simulink model "newfinal"  (R2022a)
settings: Solver=VariableStepAuto  StartTime=0.0  StopTime=time_to_simulate  RelTol=1e-3
model workspace (MAT data in the model file):
  Lm = 0.126
  Rm = 146.7889
  windingl = [0.3203609 0.3203609 0.3203609 0.000464923 0.000464923 0.000464923]
  windingr = [0.046115 0.046115 0.046115 6.692455e-05 6.692455e-05 6.692455e-05]
undefined symbols (not defined in the file): f, L1Aa, L1Ab, L1Ac, L1Ba, L1Bb, L1Bc, L1Ca, L1Cb, L1Cc, L2Aa, L2Ab, L2Ac, L2Ba, L2Bb, L2Bc, L2Ca, L2Cb, L2Cc, R1Aa, R1Ab, R1Ac, R1Ba, R1Bb, R1Bc, R1Ca, R1Cb, R1Cc, R2Aa, R2Ab, R2Ac, R2Ba, R2Bb, R2Bc, R2Ca, R2Cb, R2Cc, Sph, Ts, U1Aa, U1Ab, U1Ac, U1Ba, U1Bb, U1Bc, U1Ca, U1Cb, U1Cc, U2Aa, U2Ab, U2Ac, U2Ba, U2Bb, U2Bc, U2Ca, U2Cb, U2Cc, V1
libraries: spsBreakerLib x18, spsCurrentMeasurementLib x12, spsVoltageMeasurementLib x6, spsMultiWindingTransformerLib x3, spsGroundLib x2, spsThreePhaseParallelRLCLoadLib x1, spsThreePhaseSourceLib x1, spspowerguiLib x1
settings Model: Creator=Edwin  LastModifiedBy=Edwin
settings DebuggingCC: UnconnectedInputMsg=warning  UnconnectedOutputMsg=warning  UnconnectedLineMsg=warning
settings RTWCC: DLArmComputeVersion=19.05

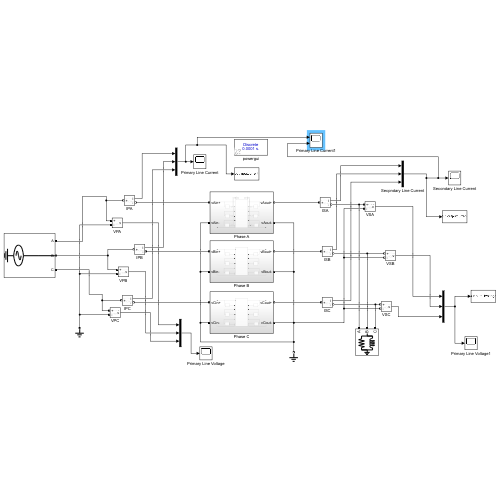
[thumbnail: Simulink's stored preview of the top-level diagram]
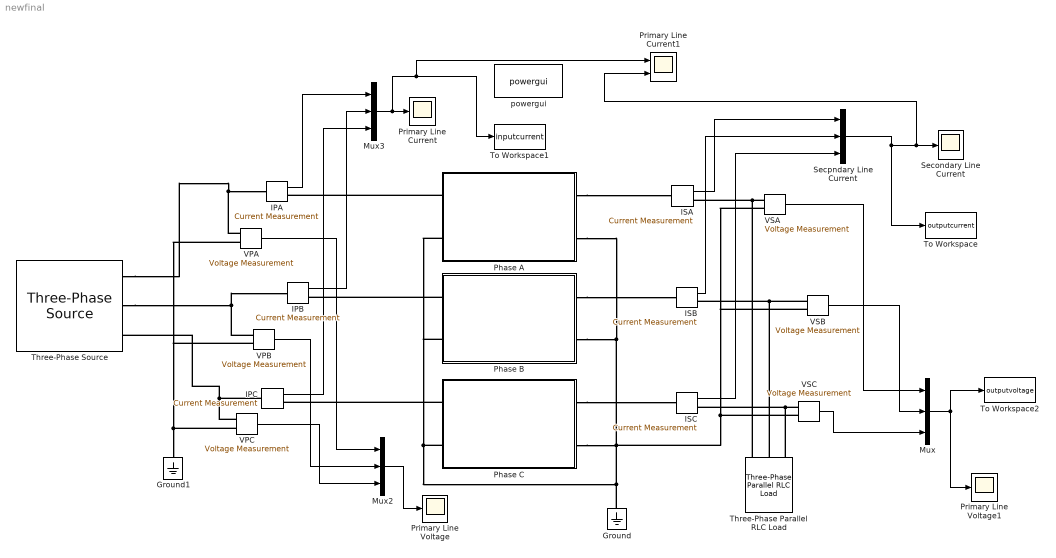
== system newfinal ==
  Ground : spsGroundLib/Ground  LConnTagsString=a
  Ground1 : spsGroundLib/Ground  LConnTagsString=a
  IPA : spsCurrentMeasurementLib/Current Measurement  PhasorSimulation=off  OutputType=Complex  PSBequivalent=0
  IPB : spsCurrentMeasurementLib/Current Measurement  PhasorSimulation=off  OutputType=Complex  PSBequivalent=0
  IPC : spsCurrentMeasurementLib/Current Measurement  PhasorSimulation=off  OutputType=Complex  PSBequivalent=0
  ISA : spsCurrentMeasurementLib/Current Measurement  PhasorSimulation=off  OutputType=Complex  PSBequivalent=0
  ISB : spsCurrentMeasurementLib/Current Measurement  PhasorSimulation=off  OutputType=Complex  PSBequivalent=0
  ISC : spsCurrentMeasurementLib/Current Measurement  PhasorSimulation=off  OutputType=Complex  PSBequivalent=0
  Mux : Mux  Inputs=3
  Mux2 : Mux  Inputs=3
  Mux3 : Mux  Inputs=3
  Phase A : Subsystem
  Phase B : Subsystem
  Phase C : Subsystem
  Primary Line Current : Scope
  Primary Line Current1 : Scope  NumInputPorts=2
  Primary Line Voltage : Scope
  Primary Line Voltage1 : Scope
  Secondary Line Current : Scope
  Secpndary Line Current : Mux  Inputs=3
  Three-Phase Parallel RLC Load : spsThreePhaseParallelRLCLoadLib/Three-Phase Parallel RLC Load  LConnTagsString=A|B|C  Configuration=Y (grounded)  NominalVoltage=V2ph  Vabc=[1e3 1e3 1e3]  Vabcp=[1e3 1e3 1e3]  NominalFrequency=f  UnbalancedPower=off  ActivePower=Pload  InductivePower=Qload  CapacitivePower=0  Pabc=[10e3 9e3 11e3]  QLabc=[100 90 110]  QCabc=[100 90 110]  Pabcp=[10e3 9e3 11e3]  QLabcp=[100 90 110]  QCabcp=[100 90 110]  Measurements=None  LoadType=constant Z
  Three-Phase Source : spsThreePhaseSourceLib/Three-Phase Source  InternalConnection=Yg  VoltagePhases=off  Voltage=V1  PhaseAngle=0  Voltage_phases=[10.5e3 10.5e3 10.5e3]/sqrt(3)  PhaseAngles_phases=[0 -120 +120]  Frequency=f  NonIdealSource=off  SpecifyImpedance=off  Resistance=0.8929  Inductance=16.58e-3  ShortCircuitLevel=100e6  BaseVoltage=25e3  XRratio=7  BusType=swing  Pref=10e3  Qref=0  Prefabc=[10e3, 10e3, 10e3]  Qrefabc=[0, 0, 0]  Qmin=-inf  Qmax=inf
  To Workspace : ToWorkspace  VariableName=outputcurrent  SampleTime=-1
  To Workspace1 : ToWorkspace  VariableName=inputcurrent  SampleTime=-1
  To Workspace2 : ToWorkspace  VariableName=outputvoltage  SampleTime=-1
  VPA : spsVoltageMeasurementLib/Voltage Measurement  PhasorSimulation=off  OutputType=Complex  PSBequivalent=0
  VPB : spsVoltageMeasurementLib/Voltage Measurement  PhasorSimulation=off  OutputType=Complex  PSBequivalent=0
  VPC : spsVoltageMeasurementLib/Voltage Measurement  PhasorSimulation=off  OutputType=Complex  PSBequivalent=0
  VSA : spsVoltageMeasurementLib/Voltage Measurement  PhasorSimulation=off  OutputType=Complex  PSBequivalent=0
  VSB : spsVoltageMeasurementLib/Voltage Measurement  PhasorSimulation=off  OutputType=Complex  PSBequivalent=0
  VSC : spsVoltageMeasurementLib/Voltage Measurement  PhasorSimulation=off  OutputType=Complex  PSBequivalent=0
  powergui : spspowerguiLib/powergui  Priority=1  SimulationMode=Discrete  SampleTime=Ts  frequency=60  Iterations=50  frequencyindice=50  Pbase=100e6  ErrMax=1e-4  UnitsV=kV  UnitsW=MW  buscounter=0  FunctionMessages=off  echomessages=off  EnableUseOfTLC=off  CurrentSourceSwitches=off  DisableSnubberDevices=off  DisableRonSwitches=off  DisableVfSwitches=off  DisplayEquations=off  AutomaticDiscreteSolvers=off  SolverType=Tustin/Backward Euler (TBE)  Interpol=off  ExternalGateDelay=off  methode=off  Ts=100  x0status=blocks  SPID=on  SwTol=0  HookPort=off  NonlinearTolerance=1e-4  nMaxIteration=100  ContinueOnMaxIteration=off  RestoreLinks=warning  ResistiveCurrentMeasurement=off  Frange=[0:2:500]  Ylog=off  Xlog=on  ShowGrid=off  save=off  variable=ZData  structure=0  ZoomFFT=off  StartTime=0.0  cycles=1  DisplayStyle=1  fundamental=60  FreqAxis=off  MaxFrequency=1000  frequencyindicesteady=1  RmsSteady=1  display=off
  wires:
  IPC/1 -> Mux3/3
  IPB/1 -> Mux3/2
  IPA/1 -> Mux3/1
  VPA/1 -> Mux2/1
  VPB/1 -> Mux2/2
  VPC/1 -> Mux2/3
  Mux3/1 -> Primary Line Current1/1, To Workspace1/1, Primary Line Current/1
  Mux2/1 -> Primary Line Voltage/1
  ISC/1 -> Secpndary Line Current/3
  ISB/1 -> Secpndary Line Current/2
  ISA/1 -> Secpndary Line Current/1
  VSA/1 -> Mux/1
  VSB/1 -> Mux/2
  VSC/1 -> Mux/3
  Secpndary Line Current/1 -> To Workspace/1, Primary Line Current1/2, Secondary Line Current/1
  Mux/1 -> To Workspace2/1, Primary Line Voltage1/1
  connections:
  Three-Phase Source/RConn1 -- VPA/LConn1 -- IPA/LConn1
  Three-Phase Source/RConn2 -- VPB/LConn1 -- IPB/LConn1
  IPC/LConn1 -- Three-Phase Source/RConn3 -- VPC/LConn1
  VPC/LConn2 -- VPA/LConn2 -- VPB/LConn2 -- Ground1/LConn1
  Phase A/LConn1 -- IPA/RConn1
  Phase B/LConn1 -- IPB/RConn1
  Phase C/LConn1 -- IPC/RConn1
  Phase A/RConn1 -- ISA/LConn1
  Phase B/RConn1 -- ISB/LConn1
  Phase C/RConn1 -- ISC/LConn1
  Ground/LConn1 -- Phase A/LConn2 -- Phase B/LConn2 -- Phase C/LConn2 -- Phase C/RConn2 -- VSC/LConn2 -- VSB/LConn2 -- VSA/LConn2 -- Phase B/RConn2 -- Phase A/RConn2
  VSC/LConn1 -- Three-Phase Parallel RLC Load/LConn3 -- ISC/RConn1
  VSB/LConn1 -- Three-Phase Parallel RLC Load/LConn2 -- ISB/RConn1
  VSA/LConn1 -- ISA/RConn1 -- Three-Phase Parallel RLC Load/LConn1

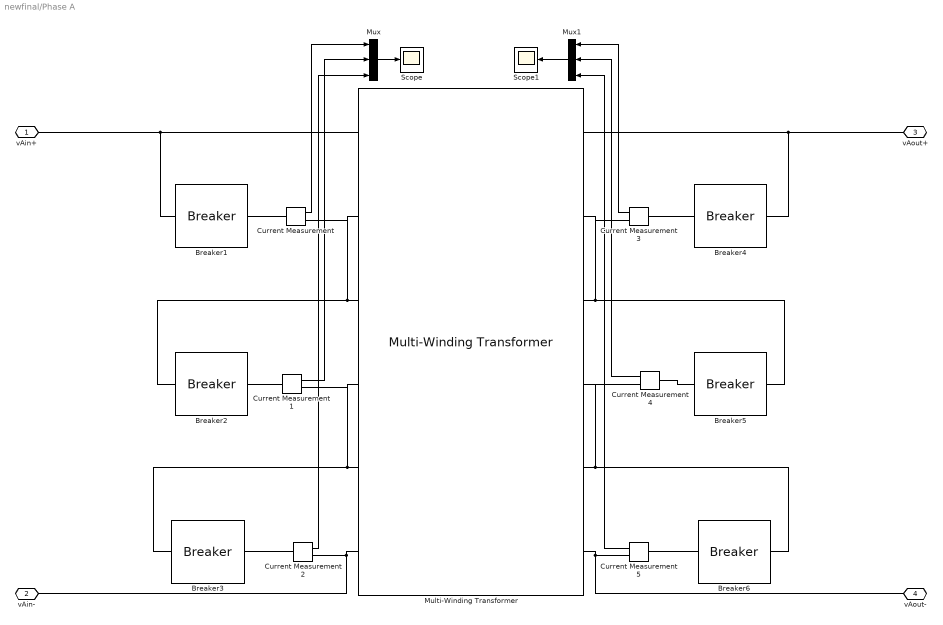
== system newfinal/Phase A ==
  Breaker1 : spsBreakerLib/Breaker  InitialState=0  SwitchingTimes=BreakerA1  External=off  BreakerResistance=0.01  SnubberResistance=1e6  SnubberCapacitance=inf  Measurements=Branch voltage and current  MoreParameters=on  NoBreakLoop=off
      settings: SourceProductBaseCode=PS
  Breaker2 : spsBreakerLib/Breaker  InitialState=0  SwitchingTimes=BreakerA2  External=off  BreakerResistance=0.01  SnubberResistance=1e6  SnubberCapacitance=inf  Measurements=Branch voltage and current  MoreParameters=on  NoBreakLoop=off
      settings: SourceProductBaseCode=PS
  Breaker3 : spsBreakerLib/Breaker  InitialState=0  SwitchingTimes=BreakerA3  External=off  BreakerResistance=0.01  SnubberResistance=1e6  SnubberCapacitance=inf  Measurements=Branch voltage and current  MoreParameters=on  NoBreakLoop=off
      settings: SourceProductBaseCode=PS
  Breaker4 : spsBreakerLib/Breaker  InitialState=0  SwitchingTimes=BreakerA4  External=off  BreakerResistance=0.01  SnubberResistance=1e6  SnubberCapacitance=inf  Measurements=Branch voltage and current  MoreParameters=on  NoBreakLoop=off
      settings: SourceProductBaseCode=PS
  Breaker5 : spsBreakerLib/Breaker  InitialState=0  SwitchingTimes=BreakerA5  External=off  BreakerResistance=0.01  SnubberResistance=1e6  SnubberCapacitance=inf  Measurements=Branch voltage and current  MoreParameters=on  NoBreakLoop=off
      settings: SourceProductBaseCode=PS
  Breaker6 : spsBreakerLib/Breaker  InitialState=0  SwitchingTimes=BreakerA6  External=off  BreakerResistance=0.01  SnubberResistance=1e6  SnubberCapacitance=inf  Measurements=Branch voltage and current  MoreParameters=on  NoBreakLoop=off
      settings: SourceProductBaseCode=PS
  Current Measurement{,1..5} (6 alike) : spsCurrentMeasurementLib/Current Measurement  PhasorSimulation=off  OutputType=Complex  PSBequivalent=0
  Multi-Winding Transformer : spsMultiWindingTransformerLib/Multi-Winding Transformer  LeftWindings=3  RightWindings=3  TappedWindings=no taps  NumberOfTaps=2  SetSaturation=off  Hysteresis=off  DataFile='hysteresis.mat'  Measurements=All measurements (V I Flux)  UNITS=SI  NominalPower=[Sph f]  NominalVoltages="[ U1Aa  U1Ab  U1Ac  U2Aa  U2Ab  U2Ac ]"  WindingResistances="[ R1Aa  R1Ab  R1Ac  R2Aa  R2Ab  R2Ac ]"  WindingInductances="[ L1Aa  L1Ab  L1Ac  L2Aa  L2Ab  L2Ac ]"  Rm=Rm  Lm=Lm  Saturation=[0 0;0.011719 56026;4.8828 70968]  SpecifyInitialFlux=off  InitialFlux=0  BreakLoop=off  DiscreteSolver=Trapezoidal iterative  DataType=on  TransfoNumber=1
      settings: SourceProductBaseCode=PS
  Mux : Mux  Inputs=3
  Mux1 : Mux  Inputs=3
  Scope : Scope
  Scope1 : Scope
  vAin+ : PMIOPort  Side=Left
  vAin- : PMIOPort  Port=2  Side=Left
  vAout+ : PMIOPort  Port=3  Side=Right
  vAout- : PMIOPort  Port=4  Side=Right
  wires:
  Current Measurement3/1 -> Mux1/1
  Current Measurement/1 -> Mux/1
  Current Measurement4/1 -> Mux1/2
  Current Measurement5/1 -> Mux1/3
  Current Measurement1/1 -> Mux/2
  Mux/1 -> Scope/1
  Current Measurement2/1 -> Mux/3
  Mux1/1 -> Scope1/1
  connections:
  Multi-Winding Transformer/LConn3 -- Breaker2/RConn1 -- Multi-Winding Transformer/LConn2 -- Current Measurement/RConn1
  Multi-Winding Transformer/RConn3 -- Multi-Winding Transformer/RConn2 -- Current Measurement3/RConn1 -- Breaker5/RConn1
  Multi-Winding Transformer/LConn5 -- Breaker3/RConn1 -- Multi-Winding Transformer/LConn4 -- Current Measurement1/RConn1
  Breaker4/RConn1 -- Multi-Winding Transformer/RConn1 -- vAout+/RConn1
  Current Measurement2/RConn1 -- vAin-/RConn1 -- Multi-Winding Transformer/LConn6
  Current Measurement5/RConn1 -- vAout-/RConn1 -- Multi-Winding Transformer/RConn6
  Multi-Winding Transformer/RConn5 -- Multi-Winding Transformer/RConn4 -- Current Measurement4/RConn1 -- Breaker6/RConn1
  Breaker1/RConn1 -- Multi-Winding Transformer/LConn1 -- vAin+/RConn1
  Current Measurement5/LConn1 -- Breaker6/LConn1
  Current Measurement2/LConn1 -- Breaker3/LConn1
  Current Measurement3/LConn1 -- Breaker4/LConn1
  Current Measurement/LConn1 -- Breaker1/LConn1
  Current Measurement4/LConn1 -- Breaker5/LConn1
  Current Measurement1/LConn1 -- Breaker2/LConn1

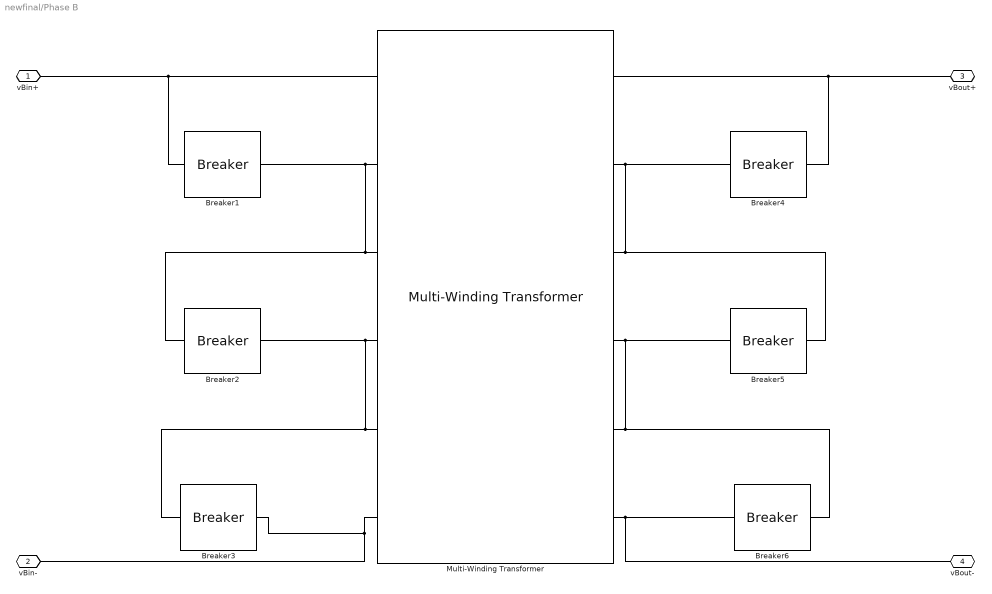
== system newfinal/Phase B ==
  Breaker1 : spsBreakerLib/Breaker  InitialState=0  SwitchingTimes=BreakerB1  External=off  BreakerResistance=0.01  SnubberResistance=1e6  SnubberCapacitance=inf  Measurements=Branch voltage and current  MoreParameters=on  NoBreakLoop=off
      settings: SourceProductBaseCode=PS
  Breaker2 : spsBreakerLib/Breaker  InitialState=0  SwitchingTimes=BreakerB2  External=off  BreakerResistance=0.01  SnubberResistance=1e6  SnubberCapacitance=inf  Measurements=Branch voltage and current  MoreParameters=on  NoBreakLoop=off
      settings: SourceProductBaseCode=PS
  Breaker3 : spsBreakerLib/Breaker  InitialState=0  SwitchingTimes=BreakerB3  External=off  BreakerResistance=0.01  SnubberResistance=1e6  SnubberCapacitance=inf  Measurements=Branch voltage and current  MoreParameters=on  NoBreakLoop=off
      settings: SourceProductBaseCode=PS
  Breaker4 : spsBreakerLib/Breaker  InitialState=0  SwitchingTimes=BreakerB4  External=off  BreakerResistance=0.01  SnubberResistance=1e6  SnubberCapacitance=inf  Measurements=Branch voltage and current  MoreParameters=on  NoBreakLoop=off
      settings: SourceProductBaseCode=PS
  Breaker5 : spsBreakerLib/Breaker  InitialState=0  SwitchingTimes=BreakerB5  External=off  BreakerResistance=0.01  SnubberResistance=1e6  SnubberCapacitance=inf  Measurements=Branch voltage and current  MoreParameters=on  NoBreakLoop=off
      settings: SourceProductBaseCode=PS
  Breaker6 : spsBreakerLib/Breaker  InitialState=0  SwitchingTimes=BreakerB6  External=off  BreakerResistance=0.01  SnubberResistance=1e6  SnubberCapacitance=inf  Measurements=Branch voltage and current  MoreParameters=on  NoBreakLoop=off
      settings: SourceProductBaseCode=PS
  Multi-Winding Transformer : spsMultiWindingTransformerLib/Multi-Winding Transformer  LeftWindings=3  RightWindings=3  TappedWindings=no taps  NumberOfTaps=2  SetSaturation=off  Hysteresis=off  DataFile='hysteresis.mat'  Measurements=All measurements (V I Flux)  UNITS=SI  NominalPower=[Sph f]  NominalVoltages="[ U1Ba  U1Bb  U1Bc  U2Ba  U2Bb  U2Bc ]"  WindingResistances="[ R1Ba  R1Bb  R1Bc  R2Ba  R2Bb  R2Bc ]"  WindingInductances="[ L1Ba  L1Bb  L1Bc  L2Ba  L2Bb  L2Bc ]"  Rm=Rm  Lm=Lm  Saturation=[0 0;0.011719 56026;4.8828 70968]  SpecifyInitialFlux=off  InitialFlux=0  BreakLoop=off  DiscreteSolver=Trapezoidal iterative  DataType=on  TransfoNumber=1
      settings: SourceProductBaseCode=PS
  vBin+ : PMIOPort  Side=Left
  vBin- : PMIOPort  Port=2  Side=Left
  vBout+ : PMIOPort  Port=3  Side=Right
  vBout- : PMIOPort  Port=4  Side=Right
  connections:
  Breaker1/LConn1 -- Multi-Winding Transformer/LConn2 -- Breaker2/RConn1 -- Multi-Winding Transformer/LConn3
  Breaker6/LConn1 -- Multi-Winding Transformer/RConn6 -- vBout-/RConn1
  Breaker4/RConn1 -- Multi-Winding Transformer/RConn1 -- vBout+/RConn1
  Multi-Winding Transformer/LConn5 -- Multi-Winding Transformer/LConn4 -- Breaker2/LConn1 -- Breaker3/RConn1
  Breaker4/LConn1 -- Multi-Winding Transformer/RConn2 -- Breaker5/RConn1 -- Multi-Winding Transformer/RConn3
  vBin-/RConn1 -- Breaker3/LConn1 -- Multi-Winding Transformer/LConn6
  Breaker5/LConn1 -- Multi-Winding Transformer/RConn4 -- Breaker6/RConn1 -- Multi-Winding Transformer/RConn5
  Breaker1/RConn1 -- Multi-Winding Transformer/LConn1 -- vBin+/RConn1

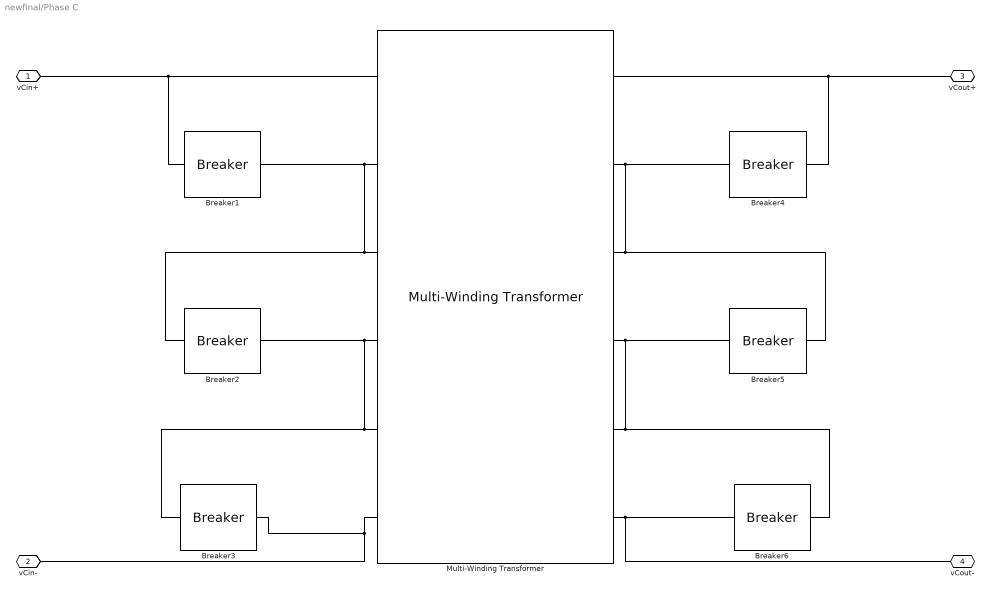
== system newfinal/Phase C ==
  Breaker1 : spsBreakerLib/Breaker  InitialState=0  SwitchingTimes=BreakerC1  External=off  BreakerResistance=0.01  SnubberResistance=1e6  SnubberCapacitance=inf  Measurements=Branch voltage and current  MoreParameters=on  NoBreakLoop=off
      settings: SourceProductBaseCode=PS
  Breaker2 : spsBreakerLib/Breaker  InitialState=0  SwitchingTimes=BreakerC2  External=off  BreakerResistance=0.01  SnubberResistance=1e6  SnubberCapacitance=inf  Measurements=Branch voltage and current  MoreParameters=on  NoBreakLoop=off
      settings: SourceProductBaseCode=PS
  Breaker3 : spsBreakerLib/Breaker  InitialState=0  SwitchingTimes=BreakerC3  External=off  BreakerResistance=0.01  SnubberResistance=1e6  SnubberCapacitance=inf  Measurements=Branch voltage and current  MoreParameters=on  NoBreakLoop=off
      settings: SourceProductBaseCode=PS
  Breaker4 : spsBreakerLib/Breaker  InitialState=0  SwitchingTimes=BreakerC4  External=off  BreakerResistance=0.01  SnubberResistance=1e6  SnubberCapacitance=inf  Measurements=Branch voltage and current  MoreParameters=on  NoBreakLoop=off
      settings: SourceProductBaseCode=PS
  Breaker5 : spsBreakerLib/Breaker  InitialState=0  SwitchingTimes=BreakerC5  External=off  BreakerResistance=0.01  SnubberResistance=1e6  SnubberCapacitance=inf  Measurements=Branch voltage and current  MoreParameters=on  NoBreakLoop=off
      settings: SourceProductBaseCode=PS
  Breaker6 : spsBreakerLib/Breaker  InitialState=0  SwitchingTimes=BreakerC6  External=off  BreakerResistance=0.01  SnubberResistance=1e6  SnubberCapacitance=inf  Measurements=Branch voltage and current  MoreParameters=on  NoBreakLoop=off
      settings: SourceProductBaseCode=PS
  Multi-Winding Transformer : spsMultiWindingTransformerLib/Multi-Winding Transformer  LeftWindings=3  RightWindings=3  TappedWindings=no taps  NumberOfTaps=2  SetSaturation=off  Hysteresis=off  DataFile='hysteresis.mat'  Measurements=All measurements (V I Flux)  UNITS=SI  NominalPower=[Sph f]  NominalVoltages="[ U1Ca  U1Cb  U1Cc  U2Ca  U2Cb  U2Cc ]"  WindingResistances="[ R1Ca  R1Cb  R1Cc  R2Ca  R2Cb  R2Cc ]"  WindingInductances="[ L1Ca  L1Cb  L1Cc  L2Ca  L2Cb  L2Cc ]"  Rm=Rm  Lm=Lm  Saturation=[0 0;0.011719 56026;4.8828 70968]  SpecifyInitialFlux=off  InitialFlux=0  BreakLoop=off  DiscreteSolver=Trapezoidal iterative  DataType=on  TransfoNumber=1
      settings: SourceProductBaseCode=PS
  vCin+ : PMIOPort  Side=Left
  vCin- : PMIOPort  Port=2  Side=Left
  vCout+ : PMIOPort  Port=3  Side=Right
  vCout- : PMIOPort  Port=4  Side=Right
  connections:
  Breaker4/RConn1 -- Multi-Winding Transformer/RConn1 -- vCout+/RConn1
  Breaker4/LConn1 -- Multi-Winding Transformer/RConn2 -- Breaker5/RConn1 -- Multi-Winding Transformer/RConn3
  Breaker5/LConn1 -- Multi-Winding Transformer/RConn4 -- Breaker6/RConn1 -- Multi-Winding Transformer/RConn5
  Multi-Winding Transformer/LConn3 -- Multi-Winding Transformer/LConn2 -- Breaker1/LConn1 -- Breaker2/RConn1
  vCin-/RConn1 -- Breaker3/LConn1 -- Multi-Winding Transformer/LConn6
  Breaker1/RConn1 -- Multi-Winding Transformer/LConn1 -- vCin+/RConn1
  Breaker2/LConn1 -- Multi-Winding Transformer/LConn4 -- Breaker3/RConn1 -- Multi-Winding Transformer/LConn5
  Breaker6/LConn1 -- Multi-Winding Transformer/RConn6 -- vCout-/RConn1
